simulink model "Self_Balance_Bot"  (R2018a)
settings: Solver=VariableStepAuto  StartTime=0.0  StopTime=20.0  RelTol=1e-3
undefined symbols (not defined in the file or in its folder): Inv
libraries: vrlib x4, simulink x1, realtime_pacer_lib x1, sharedtransform x1
settings Model: Creator=Jarvis  LastModifiedBy=Jarvis
settings SolverCC: AlgebraicLoopSolver=LineSearch

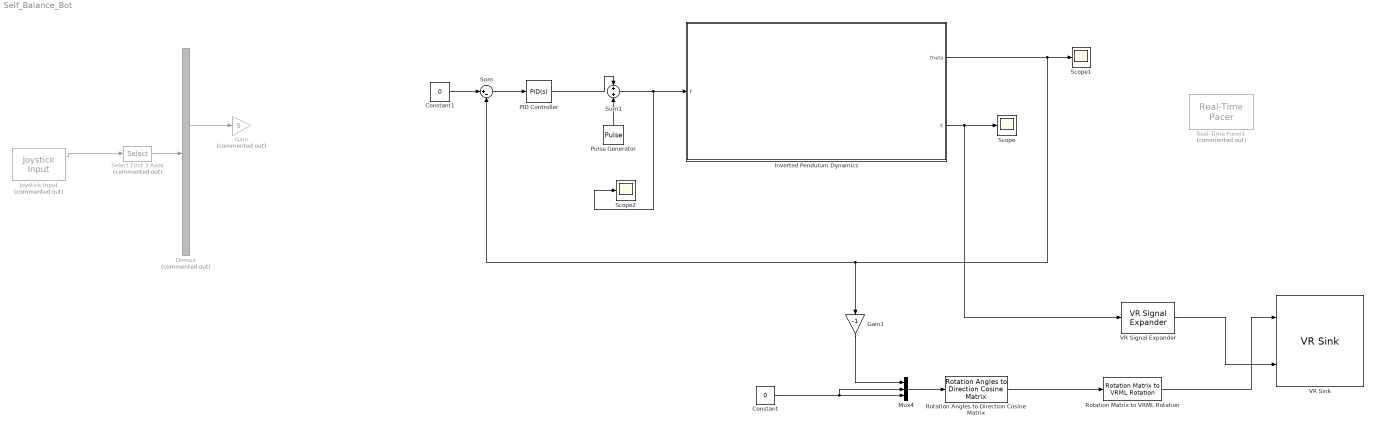
== system Self_Balance_Bot ==
  Constant : Constant  Value=0
  Constant1 : Constant  Value=0
  Demux : Demux  Commented=on
  Gain : Gain  Commented=on  Gain=5
  Gain1 : Gain  Gain=-1
  Inverted Pendulum Dynamics : Subsystem
  Joystick Input : vrlib/Joystick Input  Commented=on  joyid=1  adjustports=on  forcefeed=off
      settings: SourceProductBaseCode=VR
  Mux4 : Mux  Inputs=3
  PID Controller : simulink/Continuous/PID Controller  Controller=PID  TimeDomain=Continuous-time  SampleTime=-1  IntegratorMethod=Forward Euler  FilterMethod=Forward Euler  Form=Parallel  UseFilter=on  ControllerParametersSource=internal  P=412.302198511131  I=8600.26125585096  D=4.54400744290852  N=69679.7697369543  InitialConditionSource=internal  InitialConditionForIntegrator=0  InitialConditionForFilter=0  ExternalReset=none  LimitOutput=off  UpperSaturationLimit=inf  LowerSaturationLimit=-inf  LinearizeAsGain=on  AntiWindupMode=none  Kb=1  TrackingMode=off  Kt=1  PParamMin=[]  PParamMax=[]  IParamMin=[]  IParamMax=[]  DParamMin=[]  DParamMax=[]  NParamMin=[]  NParamMax=[]  KbParamMin=[]  KbParamMax=[]  KtParamMin=[]  KtParamMax=[]  POutMin=[]  POutMax=[]  IOutMin=[]  IOutMax=[]  DOutMin=[]  DOutMax=[]  NOutMin=[]  NOutMax=[]  KbOutMin=[]  KbOutMax=[]  KtOutMin=[]  KtOutMax=[]  IntegratorOutMin=[]  IntegratorOutMax=[]  FilterOutMin=[]  FilterOutMax=[]  SumOutMin=[]  SumOutMax=[]  SumI1OutMin=[]  SumI1OutMax=[]  SumI2OutMin=[]  SumI2OutMax=[]  SumI3OutMin=[]  SumI3OutMax=[]  SumDOutMin=[]  SumDOutMax=[]  SaturationOutMin=[]  SaturationOutMax=[]  IntegratorContinuousStateAttributes=''  IntegratorStateMustResolveToSignalObject=off  IntegratorRTWStateStorageClass=Auto  FilterContinuousStateAttributes=''  FilterStateMustResolveToSignalObject=off  FilterRTWStateStorageClass=Auto  DifferentiatorICPrevScaledInput=0  DifferentiatorOutMin=[]  DifferentiatorOutMax=[]  FilterDiffOutCoefMin=[]  FilterDiffOutCoefMax=[]  SumDenOutMin=[]  SumDenOutMax=[]  SumNumOutMin=[]  SumNumOutMax=[]  ReciprocalOutMin=[]  ReciprocalOutMax=[]  DivideOutMin=[]  DivideOutMax=[]  TunerSelectOption=Transfer Function Based (PID Tuner App)
  Pulse Generator : DiscretePulseGenerator  PulseType=Time based  Amplitude=1000  Period=1000  PulseWidth=0.001  PhaseDelay=7
  Real-Time Pacer1 : realtime_pacer_lib/Real-Time Pacer  Commented=on  simTimePerRealTime=1
  Rotation Angles to Direction Cosine Matrix : sharedtransform/Rotation Angles to Direction Cosine Matrix  rotationOrder=ZYX  aMode=aMode
      settings: SourceProductBaseCode=AE
  Rotation Matrix to VRML Rotation : vrlib/Utilities/Rotation Matrix to VRML Rotation  maxzero=1e-12
      settings: SourceProductName=Simulink 3D Animation  SourceProductBaseCode=VR
  Scope : Scope
  Scope1 : Scope
  Scope2 : Scope
  Select First 3 Axes : Selector  Commented=on  InputPortWidth=5  IndexOptions=Index vector (dialog)  Indices=[1 2 3 4]  OutputSizes=1
      settings: AttributesFormatString=(Joystick - dependent)
  Sum : Sum  Inputs=|+-
  Sum1 : Sum
  VR Signal Expander : vrlib/VR Signal Expander  outwidth=3  outidx=[1]
      settings: SourceProductName=Simulink 3D Animation  SourceProductBaseCode=VR
  VR Sink : vrlib/VR Sink  InstantiateOnLoad=on  SampleTime=0.01  ViewEnable=on  RemoteChange=off  RemoteView=off  FieldsWritten=Body.rotation.4.1.1.double#Body.translation.3.1.1.double  WorldFileName=Self_Balance_Bot.wrl  AutoView=off  VideoDimensions=[]  AllowVariableSize=off
      settings: SourceProductBaseCode=VR
  wires:
  Inverted Pendulum Dynamics/1(theta) -> Sum/2, Gain1/1, Scope1/1
  PID Controller/1 -> Sum1/1
  Pulse Generator/1 -> Sum1/2
  Constant1/1 -> Sum/1
  Sum1/1 -> Scope2/1, Inverted Pendulum Dynamics/1(F)
  Demux/2 -> Gain/1
  Gain1/1 -> Mux4/1
  Select First 3 Axes/1 -> Demux/1
  Sum/1 -> PID Controller/1
  Inverted Pendulum Dynamics/2(X) -> VR Signal Expander/1, Scope/1
  Rotation Angles to Direction Cosine Matrix/1 -> Rotation Matrix to VRML Rotation/1
  Mux4/1 -> Rotation Angles to Direction Cosine Matrix/1
  Constant/1 -> Mux4/3, Mux4/2
  Joystick Input/1 -> Select First 3 Axes/1
  VR Signal Expander/1 -> VR Sink/2
  Rotation Matrix to VRML Rotation/1 -> VR Sink/1

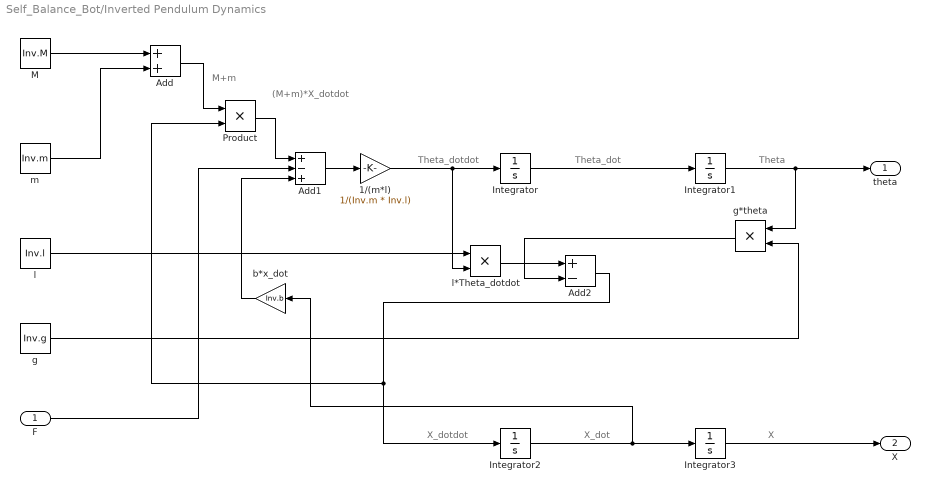
== system Self_Balance_Bot/Inverted Pendulum Dynamics ==
  note: X_dotdot
  note: Theta_dotdot
  note: M+m
  note: Theta_dot
  note: Theta
  note: X
  note: X_dot
  note: (M+m)*X_dotdot
  F : Inport
  1/(m*l) : Gain  Gain=1/(Inv.m * Inv.l)
  Add : Sum
  Add1 : Sum  Inputs=+-+
  Add2 : Sum  Inputs=+-
  Integrator{,1..3} (4 alike) : Integrator
  M : Constant  Value=Inv.M
  Product : Product
  b*x_dot : Gain  Gain=Inv.b
  g : Constant  Value=Inv.g
  g*theta : Product
  l : Constant  Value=Inv.l
  l*Theta_dotdot : Product
  m : Constant  Value=Inv.m
  theta : Outport
  X : Outport  Port=2
  wires:
  Integrator/1 -> Integrator1/1
  Integrator2/1 -> b*x_dot/1, Integrator3/1
  M/1 -> Add/1
  m/1 -> Add/2
  Add/1 -> Product/1
  F/1 -> Add1/2
  Product/1 -> Add1/1
  Add1/1 -> 1/(m*l)/1
  1/(m*l)/1 -> l*Theta_dotdot/2, Integrator/1
  Integrator1/1 -> g*theta/1, theta/1
  Integrator3/1 -> X/1
  l/1 -> l*Theta_dotdot/1
  l*Theta_dotdot/1 -> Add2/1
  g/1 -> g*theta/2
  g*theta/1 -> Add2/2
  Add2/1 -> Product/2, Integrator2/1
  b*x_dot/1 -> Add1/3
